simulink model "flattening_4_test"  (Simulink 9.0)
settings: Solver=FixedStepAuto  StartTime=0.0  StopTime=10.0  FixedStep=0.1  RelTol=1e-3  EnableMultiTasking=on
settings Model: SuppressorTable=22 serialization::archive 11 0 6 0 0 0 0 0  Creator=arnaud  LastModifiedBy=hbourbou
settings DataIOCC: LimitDataPoints=on  SignalLoggingSaveFormat=ModelDataLogs
settings OptimizationCC: ExpressionDepthLimit=2147483647
settings DebuggingCC: SolverPrmCheckMsg=warning  FcnCallInpInsideContextMsg=warning  StateNameClashWarn=warning  StrictBusMsg=Warning
settings GRTTargetCC: CombineOutputUpdateFcns=off  GRTInterface=on

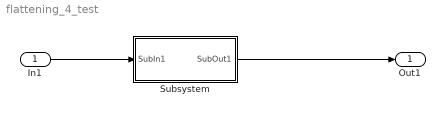
== system flattening_4_test ==
  In1 : Inport
  Subsystem : Subsystem
  Out1 : Outport
  wires:
  In1/1 -> Subsystem/1(SubIn1)
  Subsystem/1(SubOut1) -> Out1/1

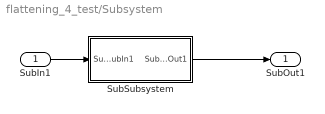
== system flattening_4_test/Subsystem ==
  SubIn1 : Inport
  SubSubsystem : Subsystem
  SubOut1 : Outport
  wires:
  SubIn1/1 -> SubSubsystem/1(SubSubIn1)
  SubSubsystem/1(SubSubOut1) -> SubOut1/1

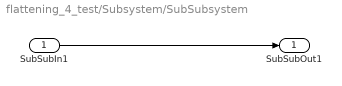
== system flattening_4_test/Subsystem/SubSubsystem ==
  SubSubIn1 : Inport
  SubSubOut1 : Outport
  wires:
  SubSubIn1/1 -> SubSubOut1/1
